simulink model "trans_16_weights"  (Simulink 6.6)
settings: Solver=VariableStepDiscrete  SolverMode=SingleTasking  StartTime=0.0  StopTime=1/10000  RelTol=1e-3
undefined symbols (not defined in the file): xlfda_numerator
libraries: xbsIndex_r4 x68, dspsrcs4 x1
settings Model: Creator=salexander  LastModifiedBy=lcrockett
settings OptimizationCC: InlineParams=on  InlineInvariantSignals=on
settings DebuggingCC: SignalResolutionControl=TryResolveAllWithWarning  MultiTaskDSMMsg=warning  MultiTaskCondExecSysMsg=none  StrictBusMsg=None
settings RTWCC: IncludeERTFirstTime=on

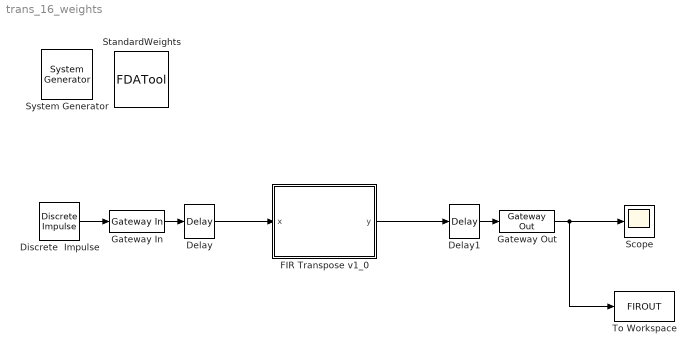
== system trans_16_weights ==
  " System Generator" : xbsIndex_r4/ System Generator  Tag=genX  SystemSampleTime=-1  xilinxfamily=virtex2p  part=xc2vp30  speed=-7  package=ff896  synthesis_tool=XST  clock_wrapper=Clock Enables  directory=./netlist  testbench=off  simulink_period=1/280e6  sysclk_period=100  dcm_input_clock_period=100  incr_netlist=off  trim_vbits=Everywhere in SubSystem  dbl_ovrd=According to Block Masks  core_generation=According to Block Masks  run_coregen=off  deprecated_control=off  eval_field=0  block_type=sysgen
      settings: block_version=8.2
  Delay : xbsIndex_r4/Delay  en=off  latency=1  dbl_ovrd=off  reg_retiming=off  block_type=delay
      settings: block_version=10.1.2
  Delay1 : xbsIndex_r4/Delay  en=off  latency=1  dbl_ovrd=off  reg_retiming=off  block_type=delay
      settings: block_version=10.1.2
  Discrete  Impulse : dspsrcs4/Discrete  Impulse  Delay=0  SampleTime=1/280e6  FrameSample=1  dataType=double  isSigned=on  wordLen=16  udDataType=sfix(16)  fracBitsMode=Best precision  numFracBits=15
  FIR Transpose v1_0 : Subsystem  mask(Transpose FIR Filter){use_emb=on, coef=xlfda_numerator('StandardWeights'), coeff_n_bits=16, coeff_f_bits=15, input_bits=8, input_f_bits=6}
      mask prompts: use_emb "Use Embedded Multipliers"; coef "Coefficients"; coeff_n_bits "Number of bits in coefficients"; coeff_f_bits "Number of fractional bits in coefficients"; input_bits "Number of bits in input"; input_f_bits "Number of fractional bits in input"
      mask help: Transpose FIR Filter
      mask init:
      | sav_gcb=gcb;
      | [bg,fg] = xlcmap('XBlock',0);
      | iPos = get_param(sav_gcb,'Position');
      | iWidth=iPos(3)-iPos(1); iHeight=iPos(4)-iPos(2);
      | iCx=iWidth/2;
      | iCy=iHeight/2;
      | [logoX, logoY] = xlogo(iPos);
      | 
      | % take the number of coefficients from the vector coef and pass it to the variable coeffs
      | coeffs = length(coef);
      | 
      | % Make sure the entered values for coeffs are positive integers
      | ncoeffs = round(sum(abs(coeffs)));
      | 
      | % find instances of mask system FIR Filter in path sav_gcb and assign to handle "update"
      | update = find_system(sav_gcb, 'lookUnderMasks', 'all', 'FollowLinks','on','masktype', 'Transpose FIR Filter');
      |     
      | % find instances of mask system Xilinx Multiplier Block in update and assign to handle "a"
      | a = find_system(update{1}, 'lookUnderMasks', 'all', 'FollowLinks','on','masktype', 'Xilinx Multiplier Block');
      | 
      | % get the number of previous coefficients
      | prev_coeffs = length(a);
      | 
      | % set disp1 and use this variable in icon tab to display string in middle of block icon
      | % disp1 = sprintf([(int2str(length(coef))) ' tap']);
      | % text(iCx/1.2,iCy/0.9,disp1);
      | % text(iCx/1.8,iCy/1.2,'Transpose FIR');
      | 
      | % issue an error if the number of coeffs entered is zero
      | if (ncoeffs < 2)
      | 	ncoeffs = prev_coeffs;
      | 	errordlg('Number of Coefficients must be at least 2')
      | end
      | 
      | % issue an error if the number of input fractional bits is greater or equal to the total number of input bits
      | if (input_f_bits >= input_bits)
      | 	errordlg('The number of fractional bits in the input must be less than the number of input bits')
      | end
      | 
      | % issue an error if the number of coefficient fractional bits is greater or equal to the total number of coefficient bits
      | if (coeff_f_bits >= coeff_n_bits)
      | 	errordlg('The number of fractional bits in the coefficients must be less than the number of coefficient bits')
      | end
      | 
      | % If number of coefficients has changed then delete all connections and blocks (except for blocks used for first two coeffs). 
      | % Then regenerate appropriate number of blocks and reconnect. Finally, reset the parameters for each block.
      | if (ncoeffs ~= prev_coeffs)
      |        
      |     % delete the connections that cannot be handled in following "for" loop
      |     delete_line(update{1}, ['AddSub' (int2str(prev_coeffs-1)) '/1'], 'y/1');
      |     
      |     % delete the connections for all blocks except the first two coefficients
      |     for i= 2:(prev_coeffs-1),
      |         delete_line(update{1}, ['Delay' int2str(i) '/1'], ['AddSub' int2str(i) '/2']);
      |         delete_line(update{1}, ['AddSub' int2str(i-1) '/1'], ['Delay' int2str(i) '/1']);
      |         delete_line(update{1}, ['Mult' int2str(i) '/1'], ['AddSub' int2str(i) '/1']);
      |         delete_line(update{1}, ['Constant' int2str(i) '/1'], ['Mult' int2str(i) '/2']);
      |         delete_line(update{1}, ['x/1'], ['Mult' int2str(i) '/1']);
      |     end
      |     
      |     % delete all blocks except those required for first two coefficients
      |     for i=2:(prev_coeffs-1),
      |         delete_block([update{1} '/Delay' int2str(i)]);
      |         delete_block([update{1} '/Constant' int2str(i)]);
      |         delete_block([update{1} '/Mult' int2str(i)]);
      |         delete_block([update{1} '/AddSub' int2str(i)]);
      |     end
      |     
      |     % regenerate appropriate number of blocks by copying existing blocks and their parameters.
      |     for i=2:(ncoeffs-1),
      |         add_block([update{1} '/Delay1'], [update{1} '/Delay' int2str(i)], 'position',[345+(i-1)*210, 250, 375+(i-1)*210, 280]);
      |         add_block([update{1} '/Mult1'], [update{1} '/Mult' int2str(i)], 'position',[340+(i-1)*210, 135, 385+(i-1)*210, 180]);
      |         add_block([update{1} '/AddSub1'], [update{1} '/AddSub' int2str(i)], 'position',[430+(i-1)*210, 230, 475+(i-1)*210, 275]);
      |         add_block([update{1} '/Constant1'], [update{1} '/Constant' int2str(i)], 'position',[205+(i-1)*210, 157, 320+(i-1)*210, 179]);
      |     end
      |     
      |     % set the position of the y output port
      |     set_param([update{1} '/' 'y'], 'Position', [520+(ncoeffs-2)*210, 250, 550+(ncoeffs-2)*210, 263]);
      |     
      |     % regenerate connections between blocks
      |     for i=2:(ncoeffs-1)
      | 		add_line(update{1}, ['x/1'], ['Mult' int2str(i) '/1'], 'autorouting', 'on');
      |         add_line(update{1}, ['Constant' int2str(i) '/1'], ['Mult' int2str(i) '/2'], 'autorouting', 'on');
      |         add_line(update{1}, ['AddSub' int2str(i-1) '/1'], ['Delay' int2str(i) '/1'], 'autorouting', 'on');
      |         add_line(update{1}, ['Delay' int2str(i) '/1'], ['AddSub' int2str(i) '/2'], 'autorouting', 'on');
      |         add_line(update{1}, ['Mult' int2str(i) '/1'], ['AddSub' int2str(i) '/1'], 'autorouting', 'on');
      |     end
      |     
      |     % connect the final AddSub block to the y output
      |     add_line(update{1}, ['AddSub' int2str(ncoeffs-1) '/1'], 'y/1', 'autorouting', 'on');
      |     
      |     % set the width of the FIR adders for each AddSub block except the first one. Also, set the weight parameter for each Constant block.
      |     for i=1:(ncoeffs-1),
      | 		set_param([update{1} '/AddSub' int2str(i)], 'n_bits', ['input_bits + coeff_n_bits + 1 + (floor(log2(' int2str(i) ')))']);
      |         % for transpose FIR the first coeff feeds the last multiplier and so on...
      |         set_param([update{1} '/Constant' int2str(i)], 'const', ['coef(' int2str(ncoeffs-i) ')']);
      |     end
      |     
      |     % Must update the first Constant block for it to take in new coefficients
      |     set_param([update{1} '/Constant'], 'const', ['coef(' int2str(ncoeffs) ')']);
      |     
      | end
      |     
      | % update the option to use embedded mults or not on all multipliers    
      | if (use_emb == 0)
      |     for i=2:ncoeffs,
      |         set_param([update{1} '/Mult' int2str(i-1)], 'use_embedded', 'off');
      |     end
      |         set_param([update{1} '/Mult'], 'use_embedded', 'off');
      | else
      |     for i=2:ncoeffs,
      |         set_param([update{1} '/Mult' int2str(i-1)], 'use_embedded', 'on');
      |     end
      |         set_param([update{1} '/Mult'], 'use_embedded', 'on');
      | end
      settings: CopyFcn=set_param(gcb, 'MaskSelfModifiable', 'on', 'LinkStatus', 'none');
      mask Display:
      | patch([0 iWidth iWidth 0],[0 0 iHeight iHeight] , bg);
      | patch(logoX,logoY , fg);
      | plot([0 0 iWidth iWidth 0], [0 iHeight iHeight 0 0]);
      | port_label('input',1,'x');
      | port_label('output',1,'y');
      | text(iCx-35, iCy, 'Transpose FIR');
  Gateway In : xbsIndex_r4/Gateway In  arith_type="Signed  (2's comp)"  n_bits=8  bin_pt=6  quantization=Truncate  overflow=Wrap  period=1/280e6  dbl_ovrd=off  timing_constraint=None  locs_specified=off  LOCs={}  block_type=gatewayin
      settings: infoedit="Gateway in block.  Converts inputs of type Simulink integer, double and fixed point to  Xilinx fixed point type.<P><P>Hardware notes:  In hardware these blocks become top level input ports."  xl_area=[0, 0, 0, 0, 0, 0, 0]  block_version=VER_STRING_GOES_HERE
  Gateway Out : xbsIndex_r4/Gateway Out  hdl_port=on  timing_constraint=None  locs_specified=off  LOCs={}  block_type=gatewayout
      settings: infoedit="Gateway out block.  Converts Xilinx fixed point inputs into ouputs of type Simulink integer, double, or fixed point.<P><P>Hardware notes:  In hardware these blocks become top level output ports or are discarded, depending on how they are configured."  xl_area=[0, 0, 0, 0, 0, 0, 0]  block_version=VER_STRING_GOES_HERE
  Scope : Scope
  StandardWeights : xbsIndex_r4/FDATool  block_type=fdatool
      settings: infoedit=FDATool  block_version=8.2
  To Workspace : ToWorkspace  VariableName=FIROUT  SampleTime=-1  SaveFormat=Array
      settings: StartFcn=close all hidden  StopFcn=doFFTplot(100e6,[FIROUT],['FIROUT'])
  wires:
  Discrete  Impulse/1 -> Gateway In/1
  Gateway Out/1 -> Scope/1, To Workspace/1
  Gateway In/1 -> Delay/1
  FIR Transpose v1_0/1(y) -> Delay1/1
  Delay/1 -> FIR Transpose v1_0/1(x)
  Delay1/1 -> Gateway Out/1

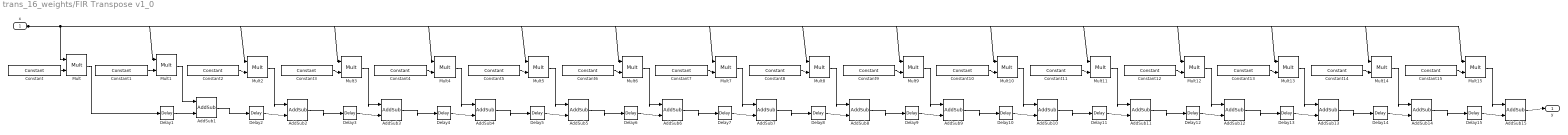
== system trans_16_weights/FIR Transpose v1_0 ==
  x : Inport
  AddSub1 : xbsIndex_r4/AddSub  mode=Addition  use_carryin=off  use_carryout=off  en=off  latency=0  precision=User Defined  arith_type="Signed  (2's comp)"  n_bits=input_bits + coeff_n_bits + 1 + (floor(log2(1)))  bin_pt=input_f_bits+coeff_f_bits  quantization=Truncate  overflow=Wrap  dbl_ovrd=off  use_behavioral_HDL=off  pipelined=off  use_rpm=on  block_type=addsub
      settings: block_version=8.2.01
  AddSub10 : xbsIndex_r4/AddSub  mode=Addition  use_carryin=off  use_carryout=off  en=off  latency=0  precision=User Defined  arith_type="Signed  (2's comp)"  n_bits=input_bits + coeff_n_bits + 1 + (floor(log2(10)))  bin_pt=input_f_bits+coeff_f_bits  quantization=Truncate  overflow=Wrap  dbl_ovrd=off  use_behavioral_HDL=off  pipelined=off  use_rpm=on  block_type=addsub
      settings: block_version=8.2.01
  AddSub11 : xbsIndex_r4/AddSub  mode=Addition  use_carryin=off  use_carryout=off  en=off  latency=0  precision=User Defined  arith_type="Signed  (2's comp)"  n_bits=input_bits + coeff_n_bits + 1 + (floor(log2(11)))  bin_pt=input_f_bits+coeff_f_bits  quantization=Truncate  overflow=Wrap  dbl_ovrd=off  use_behavioral_HDL=off  pipelined=off  use_rpm=on  block_type=addsub
      settings: block_version=8.2.01
  AddSub12 : xbsIndex_r4/AddSub  mode=Addition  use_carryin=off  use_carryout=off  en=off  latency=0  precision=User Defined  arith_type="Signed  (2's comp)"  n_bits=input_bits + coeff_n_bits + 1 + (floor(log2(12)))  bin_pt=input_f_bits+coeff_f_bits  quantization=Truncate  overflow=Wrap  dbl_ovrd=off  use_behavioral_HDL=off  pipelined=off  use_rpm=on  block_type=addsub
      settings: block_version=8.2.01
  AddSub13 : xbsIndex_r4/AddSub  mode=Addition  use_carryin=off  use_carryout=off  en=off  latency=0  precision=User Defined  arith_type="Signed  (2's comp)"  n_bits=input_bits + coeff_n_bits + 1 + (floor(log2(13)))  bin_pt=input_f_bits+coeff_f_bits  quantization=Truncate  overflow=Wrap  dbl_ovrd=off  use_behavioral_HDL=off  pipelined=off  use_rpm=on  block_type=addsub
      settings: block_version=8.2.01
  AddSub14 : xbsIndex_r4/AddSub  mode=Addition  use_carryin=off  use_carryout=off  en=off  latency=0  precision=User Defined  arith_type="Signed  (2's comp)"  n_bits=input_bits + coeff_n_bits + 1 + (floor(log2(14)))  bin_pt=input_f_bits+coeff_f_bits  quantization=Truncate  overflow=Wrap  dbl_ovrd=off  use_behavioral_HDL=off  pipelined=off  use_rpm=on  block_type=addsub
      settings: block_version=8.2.01
  AddSub15 : xbsIndex_r4/AddSub  mode=Addition  use_carryin=off  use_carryout=off  en=off  latency=0  precision=User Defined  arith_type="Signed  (2's comp)"  n_bits=input_bits + coeff_n_bits + 1 + (floor(log2(15)))  bin_pt=input_f_bits+coeff_f_bits  quantization=Truncate  overflow=Wrap  dbl_ovrd=off  use_behavioral_HDL=off  pipelined=off  use_rpm=on  block_type=addsub
      settings: block_version=8.2.01
  AddSub2 : xbsIndex_r4/AddSub  mode=Addition  use_carryin=off  use_carryout=off  en=off  latency=0  precision=User Defined  arith_type="Signed  (2's comp)"  n_bits=input_bits + coeff_n_bits + 1 + (floor(log2(2)))  bin_pt=input_f_bits+coeff_f_bits  quantization=Truncate  overflow=Wrap  dbl_ovrd=off  use_behavioral_HDL=off  pipelined=off  use_rpm=on  block_type=addsub
      settings: block_version=8.2.01
  AddSub3 : xbsIndex_r4/AddSub  mode=Addition  use_carryin=off  use_carryout=off  en=off  latency=0  precision=User Defined  arith_type="Signed  (2's comp)"  n_bits=input_bits + coeff_n_bits + 1 + (floor(log2(3)))  bin_pt=input_f_bits+coeff_f_bits  quantization=Truncate  overflow=Wrap  dbl_ovrd=off  use_behavioral_HDL=off  pipelined=off  use_rpm=on  block_type=addsub
      settings: block_version=8.2.01
  AddSub4 : xbsIndex_r4/AddSub  mode=Addition  use_carryin=off  use_carryout=off  en=off  latency=0  precision=User Defined  arith_type="Signed  (2's comp)"  n_bits=input_bits + coeff_n_bits + 1 + (floor(log2(4)))  bin_pt=input_f_bits+coeff_f_bits  quantization=Truncate  overflow=Wrap  dbl_ovrd=off  use_behavioral_HDL=off  pipelined=off  use_rpm=on  block_type=addsub
      settings: block_version=8.2.01
  AddSub5 : xbsIndex_r4/AddSub  mode=Addition  use_carryin=off  use_carryout=off  en=off  latency=0  precision=User Defined  arith_type="Signed  (2's comp)"  n_bits=input_bits + coeff_n_bits + 1 + (floor(log2(5)))  bin_pt=input_f_bits+coeff_f_bits  quantization=Truncate  overflow=Wrap  dbl_ovrd=off  use_behavioral_HDL=off  pipelined=off  use_rpm=on  block_type=addsub
      settings: block_version=8.2.01
  AddSub6 : xbsIndex_r4/AddSub  mode=Addition  use_carryin=off  use_carryout=off  en=off  latency=0  precision=User Defined  arith_type="Signed  (2's comp)"  n_bits=input_bits + coeff_n_bits + 1 + (floor(log2(6)))  bin_pt=input_f_bits+coeff_f_bits  quantization=Truncate  overflow=Wrap  dbl_ovrd=off  use_behavioral_HDL=off  pipelined=off  use_rpm=on  block_type=addsub
      settings: block_version=8.2.01
  AddSub7 : xbsIndex_r4/AddSub  mode=Addition  use_carryin=off  use_carryout=off  en=off  latency=0  precision=User Defined  arith_type="Signed  (2's comp)"  n_bits=input_bits + coeff_n_bits + 1 + (floor(log2(7)))  bin_pt=input_f_bits+coeff_f_bits  quantization=Truncate  overflow=Wrap  dbl_ovrd=off  use_behavioral_HDL=off  pipelined=off  use_rpm=on  block_type=addsub
      settings: block_version=8.2.01
  AddSub8 : xbsIndex_r4/AddSub  mode=Addition  use_carryin=off  use_carryout=off  en=off  latency=0  precision=User Defined  arith_type="Signed  (2's comp)"  n_bits=input_bits + coeff_n_bits + 1 + (floor(log2(8)))  bin_pt=input_f_bits+coeff_f_bits  quantization=Truncate  overflow=Wrap  dbl_ovrd=off  use_behavioral_HDL=off  pipelined=off  use_rpm=on  block_type=addsub
      settings: block_version=8.2.01
  AddSub9 : xbsIndex_r4/AddSub  mode=Addition  use_carryin=off  use_carryout=off  en=off  latency=0  precision=User Defined  arith_type="Signed  (2's comp)"  n_bits=input_bits + coeff_n_bits + 1 + (floor(log2(9)))  bin_pt=input_f_bits+coeff_f_bits  quantization=Truncate  overflow=Wrap  dbl_ovrd=off  use_behavioral_HDL=off  pipelined=off  use_rpm=on  block_type=addsub
      settings: block_version=8.2.01
  Constant : xbsIndex_r4/Constant  arith_type=Signed (2's comp)  const=coef(16)  n_bits=coeff_n_bits  bin_pt=coeff_f_bits  explicit_period=off  period=1  equ=P=C  opselect=C  inp2=PCIN>>17  opr=+  inp1=P  carry=CIN  dbl_ovrd=off  block_type=constant
      settings: block_version=8.2.01
  Constant1 : xbsIndex_r4/Constant  arith_type=Signed (2's comp)  const=coef(15)  n_bits=coeff_n_bits  bin_pt=coeff_f_bits  explicit_period=off  period=1  equ=P=C  opselect=C  inp2=PCIN>>17  opr=+  inp1=P  carry=CIN  dbl_ovrd=off  block_type=constant
      settings: block_version=8.2.01
  Constant10 : xbsIndex_r4/Constant  arith_type=Signed (2's comp)  const=coef(6)  n_bits=coeff_n_bits  bin_pt=coeff_f_bits  explicit_period=off  period=1  equ=P=C  opselect=C  inp2=PCIN>>17  opr=+  inp1=P  carry=CIN  dbl_ovrd=off  block_type=constant
      settings: block_version=8.2.01
  Constant11 : xbsIndex_r4/Constant  arith_type=Signed (2's comp)  const=coef(5)  n_bits=coeff_n_bits  bin_pt=coeff_f_bits  explicit_period=off  period=1  equ=P=C  opselect=C  inp2=PCIN>>17  opr=+  inp1=P  carry=CIN  dbl_ovrd=off  block_type=constant
      settings: block_version=8.2.01
  Constant12 : xbsIndex_r4/Constant  arith_type=Signed (2's comp)  const=coef(4)  n_bits=coeff_n_bits  bin_pt=coeff_f_bits  explicit_period=off  period=1  equ=P=C  opselect=C  inp2=PCIN>>17  opr=+  inp1=P  carry=CIN  dbl_ovrd=off  block_type=constant
      settings: block_version=8.2.01
  Constant13 : xbsIndex_r4/Constant  arith_type=Signed (2's comp)  const=coef(3)  n_bits=coeff_n_bits  bin_pt=coeff_f_bits  explicit_period=off  period=1  equ=P=C  opselect=C  inp2=PCIN>>17  opr=+  inp1=P  carry=CIN  dbl_ovrd=off  block_type=constant
      settings: block_version=8.2.01
  Constant14 : xbsIndex_r4/Constant  arith_type=Signed (2's comp)  const=coef(2)  n_bits=coeff_n_bits  bin_pt=coeff_f_bits  explicit_period=off  period=1  equ=P=C  opselect=C  inp2=PCIN>>17  opr=+  inp1=P  carry=CIN  dbl_ovrd=off  block_type=constant
      settings: block_version=8.2.01
  Constant15 : xbsIndex_r4/Constant  arith_type=Signed (2's comp)  const=coef(1)  n_bits=coeff_n_bits  bin_pt=coeff_f_bits  explicit_period=off  period=1  equ=P=C  opselect=C  inp2=PCIN>>17  opr=+  inp1=P  carry=CIN  dbl_ovrd=off  block_type=constant
      settings: block_version=8.2.01
  Constant2 : xbsIndex_r4/Constant  arith_type=Signed (2's comp)  const=coef(14)  n_bits=coeff_n_bits  bin_pt=coeff_f_bits  explicit_period=off  period=1  equ=P=C  opselect=C  inp2=PCIN>>17  opr=+  inp1=P  carry=CIN  dbl_ovrd=off  block_type=constant
      settings: block_version=8.2.01
  Constant3 : xbsIndex_r4/Constant  arith_type=Signed (2's comp)  const=coef(13)  n_bits=coeff_n_bits  bin_pt=coeff_f_bits  explicit_period=off  period=1  equ=P=C  opselect=C  inp2=PCIN>>17  opr=+  inp1=P  carry=CIN  dbl_ovrd=off  block_type=constant
      settings: block_version=8.2.01
  Constant4 : xbsIndex_r4/Constant  arith_type=Signed (2's comp)  const=coef(12)  n_bits=coeff_n_bits  bin_pt=coeff_f_bits  explicit_period=off  period=1  equ=P=C  opselect=C  inp2=PCIN>>17  opr=+  inp1=P  carry=CIN  dbl_ovrd=off  block_type=constant
      settings: block_version=8.2.01
  Constant5 : xbsIndex_r4/Constant  arith_type=Signed (2's comp)  const=coef(11)  n_bits=coeff_n_bits  bin_pt=coeff_f_bits  explicit_period=off  period=1  equ=P=C  opselect=C  inp2=PCIN>>17  opr=+  inp1=P  carry=CIN  dbl_ovrd=off  block_type=constant
      settings: block_version=8.2.01
  Constant6 : xbsIndex_r4/Constant  arith_type=Signed (2's comp)  const=coef(10)  n_bits=coeff_n_bits  bin_pt=coeff_f_bits  explicit_period=off  period=1  equ=P=C  opselect=C  inp2=PCIN>>17  opr=+  inp1=P  carry=CIN  dbl_ovrd=off  block_type=constant
      settings: block_version=8.2.01
  Constant7 : xbsIndex_r4/Constant  arith_type=Signed (2's comp)  const=coef(9)  n_bits=coeff_n_bits  bin_pt=coeff_f_bits  explicit_period=off  period=1  equ=P=C  opselect=C  inp2=PCIN>>17  opr=+  inp1=P  carry=CIN  dbl_ovrd=off  block_type=constant
      settings: block_version=8.2.01
  Constant8 : xbsIndex_r4/Constant  arith_type=Signed (2's comp)  const=coef(8)  n_bits=coeff_n_bits  bin_pt=coeff_f_bits  explicit_period=off  period=1  equ=P=C  opselect=C  inp2=PCIN>>17  opr=+  inp1=P  carry=CIN  dbl_ovrd=off  block_type=constant
      settings: block_version=8.2.01
  Constant9 : xbsIndex_r4/Constant  arith_type=Signed (2's comp)  const=coef(7)  n_bits=coeff_n_bits  bin_pt=coeff_f_bits  explicit_period=off  period=1  equ=P=C  opselect=C  inp2=PCIN>>17  opr=+  inp1=P  carry=CIN  dbl_ovrd=off  block_type=constant
      settings: block_version=8.2.01
  Delay{1..15} (15 alike) : xbsIndex_r4/Delay  en=off  latency=1  dbl_ovrd=off  reg_retiming=off  block_type=delay
      settings: infoedit=Hardware notes: A delay line is a chain, each link of which is an SRL16 followed by a flip-flop. If register retiming is enabled, the delay line is a chain of flip-flops.  block_version=8.2.01
  Mult{,1..15} (16 alike) : xbsIndex_r4/Mult  precision=User Defined  arith_type="Signed  (2's comp)"  n_bits=input_bits+coeff_n_bits  bin_pt=input_f_bits+coeff_f_bits  quantization=Truncate  overflow=Wrap  en=off  latency=0  dbl_ovrd=off  use_behavioral_HDL=off  use_embedded=on  opt=Speed  optimum_pipeline=off  pipeline=on  use_rpm=on  placement_style=Rectangular shape  block_type=mult
      settings: infoedit=Hardware notes: To use the internal pipeline stage of the dedicated multiplier you must select 'Pipeline for maximum performance'.  block_version=8.2.01
  y : Outport
  wires:
  Delay1/1 -> AddSub1/2
  Mult1/1 -> AddSub1/1
  Mult/1 -> Delay1/1
  Constant1/1 -> Mult1/2
  Constant/1 -> Mult/2
  x/1 -> Mult1/1, Mult/1, Mult2/1, Mult3/1, Mult4/1, Mult5/1, Mult6/1, Mult7/1, Mult8/1, Mult9/1, Mult10/1, Mult11/1, Mult12/1, Mult13/1, Mult14/1, Mult15/1
  Constant2/1 -> Mult2/2
  AddSub1/1 -> Delay2/1
  Delay2/1 -> AddSub2/2
  Mult2/1 -> AddSub2/1
  Constant3/1 -> Mult3/2
  AddSub2/1 -> Delay3/1
  Delay3/1 -> AddSub3/2
  Mult3/1 -> AddSub3/1
  Constant4/1 -> Mult4/2
  AddSub3/1 -> Delay4/1
  Delay4/1 -> AddSub4/2
  Mult4/1 -> AddSub4/1
  Constant5/1 -> Mult5/2
  AddSub4/1 -> Delay5/1
  Delay5/1 -> AddSub5/2
  Mult5/1 -> AddSub5/1
  Constant6/1 -> Mult6/2
  AddSub5/1 -> Delay6/1
  Delay6/1 -> AddSub6/2
  Mult6/1 -> AddSub6/1
  Constant7/1 -> Mult7/2
  AddSub6/1 -> Delay7/1
  Delay7/1 -> AddSub7/2
  Mult7/1 -> AddSub7/1
  Constant8/1 -> Mult8/2
  AddSub7/1 -> Delay8/1
  Delay8/1 -> AddSub8/2
  Mult8/1 -> AddSub8/1
  Constant9/1 -> Mult9/2
  AddSub8/1 -> Delay9/1
  Delay9/1 -> AddSub9/2
  Mult9/1 -> AddSub9/1
  Constant10/1 -> Mult10/2
  AddSub9/1 -> Delay10/1
  Delay10/1 -> AddSub10/2
  Mult10/1 -> AddSub10/1
  Constant11/1 -> Mult11/2
  AddSub10/1 -> Delay11/1
  Delay11/1 -> AddSub11/2
  Mult11/1 -> AddSub11/1
  Constant12/1 -> Mult12/2
  AddSub11/1 -> Delay12/1
  Delay12/1 -> AddSub12/2
  Mult12/1 -> AddSub12/1
  Constant13/1 -> Mult13/2
  AddSub12/1 -> Delay13/1
  Delay13/1 -> AddSub13/2
  Mult13/1 -> AddSub13/1
  Constant14/1 -> Mult14/2
  AddSub13/1 -> Delay14/1
  Delay14/1 -> AddSub14/2
  Mult14/1 -> AddSub14/1
  Constant15/1 -> Mult15/2
  AddSub14/1 -> Delay15/1
  Delay15/1 -> AddSub15/2
  Mult15/1 -> AddSub15/1
  AddSub15/1 -> y/1
